simulink model "simplified_powertrain"  (R2020b)
settings: Solver=FixedStepAuto  StartTime=0.0  StopTime=60  RelTol=1e-3
PreLoadFcn:
  | C_sc = 1;
StartFcn:
  | C_sc = 1;
values from neighbouring files (symbols this model uses):
  D = 0    [model_fc.m]
undefined symbols (not defined in the file or in its folder): command, DiscIntNeverNeededParam, ECMS, Flight, in, Ion, Lithium, out, w
libraries: powerlib x22, electricdrivelib x3, lib_converters x3, simulink x2, fuzblock x1, mpclib x1, re_lib x1
(part 6 of 6)

== matlab function simplified_powertrain/EMS/Management Variant/MPC/MATLAB Function ==
  settings: updateMethod=DISCRETE  sampleTime=Ts
  data: Vbatt input; Ibatt input; Ibatt_out input; Ibatt_1 output; Ifc_out input; Vpv input; Ipv input; Ipv_out input; Pload input; Vdc input; Vdc_wanted input; Pout input; Ibatt_2 output; Ibatt_3 output; IO_batt_conv output; IO_batt_conv_value input; Ifc_boost input; Vfc input
function [Ibatt_1, Ibatt_2, Ibatt_3,  IO_batt_conv] = fcn(Vbatt, Ibatt,Ibatt_out, Ifc_out, Vpv, Ipv, Ipv_out,Pload,Vdc,Vdc_wanted, Pout, IO_batt_conv_value, Ifc_boost, Vfc)
    %% Part - 1
    %     FC = Vfc * Ifc_boost;
    %     FC = Vfc * Ifc_in;
    %     FC = Vdc_wanted * Ifc_out;
    FC = Vdc * Ifc_out;
    
    %     PV = Vpv * Ipv_boost;
%         PV = Vpv * Ipv; % stable pv panel but not good
    %     PV = Vdc_wanted * Ipv_out;
    PV = Vdc * Ipv_out; % marche mieux avec celui ci mais pv pas au max
    
    %     Batt = Vbatt * Ibatt;
    Batt = Vdc * Ibatt_out;
    
    %     Ibatt_1 = (Pload - FC - PV)/Vdc_wanted;
    %     Ibatt_1 = (Pload - FC - PV)/Vdc;
    Ibatt_1 = (Pload - FC - PV - Batt)/Vdc;
    %     Ibatt_1 = -10;
    
    %% Part - 2
    Ibatt_2 = Pload - Pout;
    
    %% Part - 3
    Ibatt_3 = Vdc_wanted - Vdc;
    
    %% Activate conv
    IO_batt_conv = IO_batt_conv_value;
end

== matlab function simplified_powertrain/EMS/Management Variant/MPC/MATLAB Function1 ==
  settings: updateMethod=DISCRETE  sampleTime=Ts
  data: current_comm input; conv output; Pload input; Vbus_required input; current_command output; V_batt_conv output
function [conv, current_command,V_batt_conv] = fcn(current_comm, Pload, Vbus_required)
    if current_comm < 0
        conv = 1;
        V_batt_conv = Vbus_required; % (55)
    else
        conv = 0;
        V_batt_conv = Vbus_required;
    end
%     V_batt_conv = 120;
    current_command = current_comm;
end

%     if Pload == 0 || current_comm < 0
%         conv = 1;
%         V_batt_conv = 50;
%     else
%         conv = 0;
%         V_batt_conv = Vbus_required;
%     end
%     current_command = current_comm;

== matlab function simplified_powertrain/EMS/Management Variant/MPC/PV - FC - control ==
  settings: updateMethod=DISCRETE  sampleTime=Ts
  data: Time input; Vdc_command input; Vfc input; Ifc_in input; Vbatt input; Ibatt_in input; Vpv input; Ifc output; Vfc_conv output; IO_fc_conv output; Pload input; Ipv_in input; SOC input; Ipv output; Vpv_conv output; IO_pv_conv output; Ipvout input; Vdc_real input; Pout_real input; Control_pv output; IO_pv_conv_value input; IO_fc_conv_value input; Control_pv_choose_var input; BATT_SOC input
function [Ifc,Vfc_conv,IO_fc_conv,Ipv,Vpv_conv,IO_pv_conv,Control_pv] = ...
        fcn(Time, Vdc_command,Vfc,Ifc_in, Vbatt, Ibatt_in, Vpv, Pload, ...
        Ipv_in, SOC, Ipvout, Vdc_real, Pout_real, IO_pv_conv_value, ...
        IO_fc_conv_value, Control_pv_choose_var, BATT_SOC)
    
%     Degradation-Conscious Equivalent Consumption Minimization Strategy for a Fuel Cell Hybrid System
    %% PV - MPPT P&O algo in Cascade control
    % Get previous values for the MPPT algo in Cascade control
    persistent Ppv_pre Ppv_w_pre;
    dataType = 'double';
    if isempty(Ppv_pre)
        Ppv_pre=0;
        Ppv_w_pre = 200;
    end
    
    
    % Set the control mode
    if Control_pv_choose_var == 0 % Auto
        Control_pv = 2; % 1 = MPPT | 2 = Cascade Control
    else
        Control_pv = Control_pv_choose_var;
    end
    
    
    Ppv_out = Ipvout*Vdc_real;
    Ppv_in = Ipv_in*Vpv;
    Delta_PV = 0.5;
    Ppv_wanted = Ppv_in;
    
    if Control_pv == 2 % Cascade control
        if mod(Time,2e-4) == 0
            if Ppv_in < Ppv_pre
                Ppv_wanted  = Ppv_in - Delta_PV;
            end
            if Ppv_in > Ppv_pre
                Ppv_wanted  = Ppv_in + Delta_PV;
            end
        end
        if Ppv_out < 0
            Ppv_wanted = 180;
        end
        
        Ipv = Ppv_wanted/Vpv;
    else
        Ipv = 0;
    end
    
    % Converter wanter output voltage
    Vpv_conv = Vdc_command;
    
    
    % PV converter operates ?
    IO_pv_conv = IO_pv_conv_value;
    
    
    % Set the values for the next loop
    Ppv_pre = Ppv_in;
    Ppv_w_pre = Ppv_wanted;
    
    
    
    
    %% FC - control
    % FC converter operates ?
    IO_fc_conv = IO_fc_conv_value;
    
    %% D-ECMS:
%     Degradation-Conscious Equivalent Consumption Minimization Strategy for a Fuel Cell Hybrid System
    Pbatt_min=-150; Pbatt_max=800;
    SOC_min=60; SOC_max=90;
    Pfc_min=400;Pfc_max=1100;
    
    %define Matrix Aeq
    Aeq=[0 1 0;1 0 1];
    
    %define Matrix beq
    mu=0.6;
    beq=[1-2*mu*((SOC-0.5*(SOC_max+SOC_min))/(SOC_max+SOC_min)); Pload-Ppv_out];
    
    %define boundary conditions
    lb=[Pfc_min, 0, Pbatt_min];
    ub=[Pfc_max, 100, Pbatt_max];
    
    %define initial conditions
    x0=[1000, 0.1, 500];
    
    options = optimoptions('fmincon','Algorithm','sqp',...
        'Display','off','MaxFunctionEvaluations',500,'MaxIterations',100);
    [y,fval] = fmincon(@(x)decms(x,Vfc,Ifc_in,Ibatt_in,SOC),x0,[],[],Aeq,beq,lb,ub,[],options);
    
    Pfc=y(1); Pbatt=y(3); alpha=y(2);
    
    
    % Ifc command
    Ifc = Pfc/Vfc;
    
    % Converter wanted output voltage
    Vfc_conv = Vdc_command;
    if Ifc_in < Ifc
        Vfc_conv = 100;
    end
    
    
function f = decms(x,Vfc,Ifc_in,Ibatt_in,SOC)
    DT=200e-3;
    do = 0.5e-4;
    alpha = 4;
    FCcost = 525;
    Hcost = 2;
    BATcost = 640;
    Pfc_nom = 1000;
    Q = 15;
    dfc = (do/3600)*(1+alpha/(Pfc_nom^2)*(Vfc*Ifc_in-Pfc_nom)^2);
    dbat = (1/Q)*abs(weight_func_1(SOC)*weight_func_2(Ibatt_in)*Ibatt_in);
    mfc_deg = dfc * FCcost / Hcost;
    mbat_deg = dbat * BATcost / Hcost;
    f = (x(1)+x(2)*x(3)+ mfc_deg + mbat_deg)*DT;
    
function out = weight_func_1(SOC)
    out = 1+3.25*(1-SOC)^2;
    
function out = weight_func_2(Ibatt)
    Ibatt_nom = 2;
    if Ibatt >= 0
        out = 1+0.45*Ibatt/Ibatt_nom;
    else
        out = 1+0.55*abs(Ibatt)/Ibatt_nom;
    end

== matlab function simplified_powertrain/MATLAB Function ==
  data: ep output; ev output; time input; error_power output; Prequired input; Preal input; Vbus_required input; Vbus_real input; error_voltage output
function [ep,ev,error_power, error_voltage] = fcn(time, Prequired, Preal, Vbus_required, Vbus_real)
    ep = (Preal-Prequired)^2;
    ev = (Vbus_real-Vbus_required)^2;
    
    error_power = 100*abs(Preal-Prequired)/abs(Prequired);
    error_voltage = 100*abs(Vbus_real-Vbus_required)/Vbus_required;
end

== matlab function simplified_powertrain/EMS/Management Variant/SMC/MATLAB Function1 ==
  settings: updateMethod=DISCRETE  sampleTime=Ts
  data: current_comm input; conv output; Pload input; Vbus_required input; current_command output; V_batt_conv output
function [conv, current_command,V_batt_conv] = fcn(current_comm, Pload, Vbus_required)
    if current_comm < 0
        conv = 1;
        V_batt_conv = Vbus_required; % (55)
    else
        conv = 0;
        V_batt_conv = Vbus_required;
    end
%     V_batt_conv = 120;
    current_command = current_comm;
end

%     if Pload == 0 || current_comm < 0
%         conv = 1;
%         V_batt_conv = 50;
%     else
%         conv = 0;
%         V_batt_conv = Vbus_required;
%     end
%     current_command = current_comm;

== matlab function simplified_powertrain/PEMFC matfunc/MATLAB Function ==
  data: Ifc input; E output; P_H2 input; P_O2 input; T input; Water_content input; delta_m input; Nfc input; E_Ner output; E_act output; E_ohm output; E_con output; U_H2 output; U_O2 output; Rohm output
function [E,E_Ner,E_act,E_ohm,E_con,U_H2,U_O2,Rohm] = fcn(Ifc,P_H2,P_O2,T,Water_content,delta_m, Nfc)
    R = 8.3145;
    Pstd = 101325;
    nF = 2*96485;
    
%     %% The operating temperature can vary depending on the ambient temp:
%     T = 3+13*exp(0.03*Ta);

    if Ifc <0
        Ifc = 40;
    end
    %% Saturation at start
    if -1.87e-4*log(Ifc) > 0
        k = 0;
    else
        if -1.87e-4*log(Ifc) < -1.2
            k = -1.2;
        else
            k = -1.87e-4*log(Ifc);
        end
    end
    %% Nernst Voltage
    % Pressure not in Pa ?
    E_Ner = 1.229 + (T-298.15) * (-0.85e-3) + T*R/nF * log(P_H2*P_O2^0.5);
    
    %% Activation loss
    % Pressure not in Pa ?
    CO2 = (P_O2/(5.08e6))*exp(498/T);
    CH2 = (P_H2/(1.09e6))*exp(-77/T);
    E_act=-0.9514 + T * (2.86e-3+2e-4*log(200)+4.3e-5*log(CH2)+7.4e-5*log(CO2)+k);
    
    %% Ohmic loss
    E_ohm = - Ifc*(delta_m/((Water_content*5.139e-3-3.26e-3)*exp(1268*(1/303-1/T))));
    
    %% Ohmic resistance
    Rohm = delta_m / (0.005139*Water_content-0.00326)*exp(1268*(1/303-1/T));
    
    %% Concentration loss
    if T>= 312.15
        E_con = (1.1e-4-1.2e-6*(T-273.15))*exp(8*Ifc/40);
    else
        E_con = (3.3e-3-8.2e-5*(T-273.15))*exp(8*Ifc/40);
    end
    
    
    %% Output voltage
    E = Nfc*(E_Ner + E_act + E_ohm - E_con);
    
    
    %% Fuel utilization
    U_H2 = 60000*Ifc*R*T*Nfc/(nF*1.16*1*0.9995*Pstd);
    
    %% Air utilization
    U_O2 = 60000*Ifc*R*T*Nfc/(2*nF*0.0181*1*0.21*Pstd);
end
